simulink model "TBRe19_ECU_1_Brake_Pressure_Conversion"  (R2017b)
settings: Solver=FixedStepDiscrete  StartTime=0.0  StopTime=inf  FixedStep=0.0001  RelTol=1e-3
PostLoadFcn:
  | model_init();
libraries: simulink x17
(part 7 of 7)

== system TBRe19_ECU_1_Brake_Pressure_Conversion/MainTask/Vehicle_Functionality_Layer/Drive_Function/Throttle_withBoost ==
  note: Throttle to torque map -
      | - What percentage of max torque to request based on throttle
      | - Needs adjusting (possibly)
  note: Max torque request to motor (at 100% throttle) under normal operation
  note: Max torque request to motor (at 100% throttle) in boost mode
  note: only acts on down press
  Throttle : Inport
  Button : Inport  Port=2
  BoostActive : Switch  Criteria=u2 ~= 0  OutDataTypeStr=int16
  Delay : Delay  DelayLength=1  InitialCondition=0
  Divide1 : Product  Inputs=**
  Divide3 : Product  Inputs=**
  ModeChange : Logic  Operator=XOR  AllPortsSameDT=off  OutDataTypeStr=boolean
  NOT : Logic  Operator=NOT  AllPortsSameDT=off  OutDataTypeStr=boolean
  RisingEdgeDet : Logic  AllPortsSameDT=off  OutDataTypeStr=boolean
  Throttle_Torque_Map_% : Lookup_n-D  NumberOfTableDimensions=1  BreakpointsForDimension1=[0,30,75,100]  Table=[0,5,50,100]  ExtrapMethod=Clip  UseLastTableValue=on  InternalRulePriority=Speed  OutDataTypeStr=int16  RndMeth=Simplest  InputSameDT=on
  UsbRx : S-Function  FunctionName=NsiUsb_Rx  Parameters=signame,sigtype,resolution,offset,unite,value,is_trigger  SFunctionDeploymentMode=off  EnableBusSupport=off  mask(MUXlink Usb Rx){signame=Max_Torque_Std, sigtype=Unsigned Byte, resolution=1, offset=0.01, unite=Nm, value=120, is_trigger=off}
      mask prompts: signame "Signal name :"; sigtype "Signal type :"; resolution "Resolution :"; offset "Offset :"; unite "Unit :"; value "Default value :"; is_trigger "Is trigger ?"
      mask help: Receive a frame on the USB Channel.
      mask init:
      | NsiUsb_Rx_InitializationFcn();
      settings: OpenFcn=NsiUsb_Rx_OpenFcn();
      mask Help:
      | eval('block=get_param(gcb, ''RTWdata'');')
      | web([docroot '\toolbox\MUXlink\html\blocks/' block.MUXlink_BlockType '.html'])
      mask Callback signame: NsiUsb_Rx_ApplyFcn(1);
      mask TypeOptions sigtype: Boolean | Signed Byte | Unsigned Byte | Signed Word | Unsigned Word | Signed Double Word | Unsigned Double Word | Single Float | Double Float
      mask Callback sigtype: NsiUsb_Rx_ApplyFcn(2);
      mask Callback resolution: NsiUsb_Rx_ApplyFcn(3);
      mask Callback offset: NsiUsb_Rx_ApplyFcn(4);
      mask Callback unite: NsiUsb_Rx_ApplyFcn(5);
      mask Callback value: NsiUsb_Rx_ApplyFcn(6);
      mask Callback is_trigger: NsiUsb_Rx_ApplyFcn(7);
      mask Display: image(imread('nsi.bmp'));text(0.5, 0.2, 'USB Rx', 'horizontalAlignment', 'center', 'verticalAlignment', 'base');plot([0.05 0.05 0.05 0.05 0.05 0.05 0.05 0.05 0.05 0.05]);port_label('output',1, 'Max_Torque_Std');
  UsbRx1 : S-Function  FunctionName=NsiUsb_Rx  Parameters=signame,sigtype,resolution,offset,unite,value,is_trigger  SFunctionDeploymentMode=off  EnableBusSupport=off  mask(MUXlink Usb Rx){signame=Max_Torque_Boost, sigtype=Unsigned Byte, resolution=1, offset=0.01, unite=Nm, value=240, is_trigger=off}
      mask prompts: signame "Signal name :"; sigtype "Signal type :"; resolution "Resolution :"; offset "Offset :"; unite "Unit :"; value "Default value :"; is_trigger "Is trigger ?"
      mask help: Receive a frame on the USB Channel.
      mask init:
      | NsiUsb_Rx_InitializationFcn();
      settings: OpenFcn=NsiUsb_Rx_OpenFcn();
      mask Help:
      | eval('block=get_param(gcb, ''RTWdata'');')
      | web([docroot '\toolbox\MUXlink\html\blocks/' block.MUXlink_BlockType '.html'])
      mask Callback signame: NsiUsb_Rx_ApplyFcn(1);
      mask TypeOptions sigtype: Boolean | Signed Byte | Unsigned Byte | Signed Word | Unsigned Word | Signed Double Word | Unsigned Double Word | Single Float | Double Float
      mask Callback sigtype: NsiUsb_Rx_ApplyFcn(2);
      mask Callback resolution: NsiUsb_Rx_ApplyFcn(3);
      mask Callback offset: NsiUsb_Rx_ApplyFcn(4);
      mask Callback unite: NsiUsb_Rx_ApplyFcn(5);
      mask Callback value: NsiUsb_Rx_ApplyFcn(6);
      mask Callback is_trigger: NsiUsb_Rx_ApplyFcn(7);
      mask Display: image(imread('nsi.bmp'));text(0.5, 0.2, 'USB Rx', 'horizontalAlignment', 'center', 'verticalAlignment', 'base');plot([0.05 0.05 0.05 0.05 0.05 0.05 0.05 0.05 0.05 0.05]);port_label('output',1, 'Max_Torque_Boost');
  prvCheck : Delay  DelayLength=1  InitialCondition=0
  Throttle_Request : Outport
  Boost_On : Outport  Port=2
  wires:
  ModeChange/1 -> Boost_On/1, BoostActive/2, Delay/1
  Throttle/1 -> Throttle_Torque_Map_%/1
  Throttle_Torque_Map_%/1 -> Divide3/1, Divide1/2  "Throttle_Request"
  Divide3/1 -> BoostActive/3
  BoostActive/1 -> Throttle_Request/1
  UsbRx1/1 -> Divide1/1
  Divide1/1 -> BoostActive/1
  UsbRx/1 -> Divide3/2
  RisingEdgeDet/1 -> ModeChange/1
  NOT/1 -> RisingEdgeDet/2
  prvCheck/1 -> NOT/1
  Delay/1 -> ModeChange/2
  Button/1 -> RisingEdgeDet/1, prvCheck/1

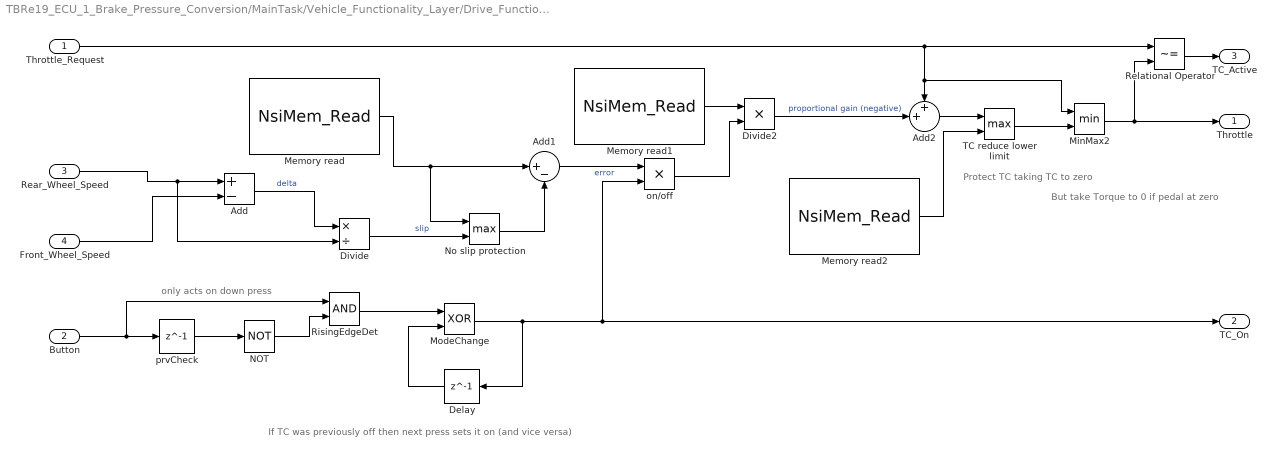
== system TBRe19_ECU_1_Brake_Pressure_Conversion/MainTask/Vehicle_Functionality_Layer/Drive_Function/Traction Control ==
  note: But take Torque to 0 if pedal at zero
  note: Protect TC taking TC to zero
  note: If TC was previously off then next press sets it on (and vice versa)
  note: only acts on down press
  Throttle_Request : Inport
  "Button " : Inport  Port=2
  Rear_Wheel_Speed : Inport  Port=3
  Front_Wheel_Speed : Inport  Port=4
  Add : Sum  Inputs=+-
  Add1 : Sum  Inputs=|+-
  Add2 : Sum  Inputs=++|
  Delay : Delay  DelayLength=1  InitialCondition=0
  Divide : Product  Inputs=*/
  Divide2 : Product  Inputs=**
  Memory read : S-Function  FunctionName=NsiMem_Read  Parameters=name_var,type_var,size_var,tunable_var  SFunctionDeploymentMode=off  EnableBusSupport=off  mask(Memory read){name_var=Target_Slip_Ratio, type_var=Single Float, size_var=1, tunable_var=on}
      mask prompts: name_var "Variable name :"; type_var "Type :"; size_var "Dim of table :"; tunable_var "Is Tunable By USB?"
      mask help: Reads current value of variable memory declared in the configurator block in calibration page.
      mask init:
      | NsiMem_Read_InitializationFcn();
      settings: OpenFcn=NsiMem_Read_OpenFcn();
      mask Help:
      | eval('block=get_param(gcb, ''RTWdata'');')
      | web([docroot '\toolbox\MUXlink\html\blocks/' block.MUXlink_BlockType '.html'])
      mask TypeOptions name_var: Gearing_Ratio | Wheel_Size | Brake1_High | Brake2_High | Accel1_High | Accel2_High | Brake1_Low | Brake2_Low | Accel1_Low | Accel2_Low | Max_Torque_Std | Max_Torque_Boost | MCU_Ignition | LV_Low_Voltage_Warning | MCUMotor_Temp_Warning | Target_Slip_Ratio | TC_P_Gain | MinTC_Torque | Max_Regen
      mask Callback name_var: NsiMem_Read_ApplyFcn(1);
      mask TypeOptions type_var: Boolean | Signed Byte | Unsigned Byte | Signed Word | Unsigned Word | Signed Double Word | Unsigned Double Word | Single Float | Double Float
      mask Callback type_var: NsiMem_Read_ApplyFcn(2);
      mask Callback size_var: NsiMem_Read_ApplyFcn(3);
      mask Callback tunable_var: NsiMem_Read_ApplyFcn(4);
      mask Display: image(imread('nsi.bmp'));text(0.5, 0.35, 'Target_Slip_Ratio', 'horizontalAlignment', 'center', 'verticalAlignment', 'base');plot([0.05 0.05 0.05 0.05 0.05 0.05 0.05 0.05 0.05 0.05]);port_label('output', 1, 'Read');
  Memory read1 : S-Function  FunctionName=NsiMem_Read  Parameters=name_var,type_var,size_var,tunable_var  SFunctionDeploymentMode=off  EnableBusSupport=off  mask(Memory read){name_var=TC_P_Gain, type_var=Unsigned Byte, size_var=1, tunable_var=on}
      mask prompts: name_var "Variable name :"; type_var "Type :"; size_var "Dim of table :"; tunable_var "Is Tunable By USB?"
      mask help: Reads current value of variable memory declared in the configurator block in calibration page.
      mask init:
      | NsiMem_Read_InitializationFcn();
      settings: OpenFcn=NsiMem_Read_OpenFcn();
      mask Help:
      | eval('block=get_param(gcb, ''RTWdata'');')
      | web([docroot '\toolbox\MUXlink\html\blocks/' block.MUXlink_BlockType '.html'])
      mask TypeOptions name_var: Gearing_Ratio | Wheel_Size | Brake1_High | Brake2_High | Accel1_High | Accel2_High | Brake1_Low | Brake2_Low | Accel1_Low | Accel2_Low | Max_Torque_Std | Max_Torque_Boost | MCU_Ignition | LV_Low_Voltage_Warning | MCUMotor_Temp_Warning | Target_Slip_Ratio | TC_P_Gain | MinTC_Torque | Max_Regen
      mask Callback name_var: NsiMem_Read_ApplyFcn(1);
      mask TypeOptions type_var: Boolean | Signed Byte | Unsigned Byte | Signed Word | Unsigned Word | Signed Double Word | Unsigned Double Word | Single Float | Double Float
      mask Callback type_var: NsiMem_Read_ApplyFcn(2);
      mask Callback size_var: NsiMem_Read_ApplyFcn(3);
      mask Callback tunable_var: NsiMem_Read_ApplyFcn(4);
      mask Display: image(imread('nsi.bmp'));text(0.5, 0.35, 'TC_P_Gain', 'horizontalAlignment', 'center', 'verticalAlignment', 'base');plot([0.05 0.05 0.05 0.05 0.05 0.05 0.05 0.05 0.05 0.05]);port_label('output', 1, 'Read');
  Memory read2 : S-Function  FunctionName=NsiMem_Read  Parameters=name_var,type_var,size_var,tunable_var  SFunctionDeploymentMode=off  EnableBusSupport=off  mask(Memory read){name_var=MinTC_Torque, type_var=Unsigned Byte, size_var=1, tunable_var=on}
      mask prompts: name_var "Variable name :"; type_var "Type :"; size_var "Dim of table :"; tunable_var "Is Tunable By USB?"
      mask help: Reads current value of variable memory declared in the configurator block in calibration page.
      mask init:
      | NsiMem_Read_InitializationFcn();
      settings: OpenFcn=NsiMem_Read_OpenFcn();
      mask Help:
      | eval('block=get_param(gcb, ''RTWdata'');')
      | web([docroot '\toolbox\MUXlink\html\blocks/' block.MUXlink_BlockType '.html'])
      mask TypeOptions name_var: Gearing_Ratio | Wheel_Size | Brake1_High | Brake2_High | Accel1_High | Accel2_High | Brake1_Low | Brake2_Low | Accel1_Low | Accel2_Low | Max_Torque_Std | Max_Torque_Boost | MCU_Ignition | LV_Low_Voltage_Warning | MCUMotor_Temp_Warning | Target_Slip_Ratio | TC_P_Gain | MinTC_Torque | Max_Regen
      mask Callback name_var: NsiMem_Read_ApplyFcn(1);
      mask TypeOptions type_var: Boolean | Signed Byte | Unsigned Byte | Signed Word | Unsigned Word | Signed Double Word | Unsigned Double Word | Single Float | Double Float
      mask Callback type_var: NsiMem_Read_ApplyFcn(2);
      mask Callback size_var: NsiMem_Read_ApplyFcn(3);
      mask Callback tunable_var: NsiMem_Read_ApplyFcn(4);
      mask Display: image(imread('nsi.bmp'));text(0.5, 0.35, 'MinTC_Torque', 'horizontalAlignment', 'center', 'verticalAlignment', 'base');plot([0.05 0.05 0.05 0.05 0.05 0.05 0.05 0.05 0.05 0.05]);port_label('output', 1, 'Read');
  MinMax2 : MinMax  Inputs=2
  ModeChange : Logic  Operator=XOR  AllPortsSameDT=off  OutDataTypeStr=boolean
  NOT : Logic  Operator=NOT  AllPortsSameDT=off  OutDataTypeStr=boolean
  No slip protection : MinMax  Function=max  Inputs=2
  Relational Operator : RelationalOperator  Operator=~=  OutDataTypeStr=boolean  RndMeth=Simplest
  RisingEdgeDet : Logic  AllPortsSameDT=off  OutDataTypeStr=boolean
  TC reduce lower limit : MinMax  Function=max  Inputs=2
  on/off : Product  Inputs=**
  prvCheck : Delay  DelayLength=1  InitialCondition=0
  Throttle : Outport
  TC_On : Outport  Port=2
  TC_Active : Outport  Port=3
  wires:
  Rear_Wheel_Speed/1 -> Divide/2, Add/1
  Front_Wheel_Speed/1 -> Add/2
  Add/1 -> Divide/1  "delta"
  Divide/1 -> No slip protection/2  "slip"
  No slip protection/1 -> Add1/2
  Memory read/1 -> No slip protection/1, Add1/1
  Add1/1 -> on/off/1  "error"
  on/off/1 -> Divide2/2
  Memory read1/1 -> Divide2/1
  Divide2/1 -> Add2/2  "proportional gain (negative)"
  Throttle_Request/1 -> Relational Operator/1, MinMax2/1, Add2/1
  Add2/1 -> TC reduce lower limit/1
  NOT/1 -> RisingEdgeDet/2
  Delay/1 -> ModeChange/2
  ModeChange/1 -> on/off/2, TC_On/1, Delay/1
  prvCheck/1 -> NOT/1
  "Button "/1 -> RisingEdgeDet/1, prvCheck/1
  RisingEdgeDet/1 -> ModeChange/1
  TC reduce lower limit/1 -> MinMax2/2
  Memory read2/1 -> TC reduce lower limit/2
  MinMax2/1 -> Relational Operator/2, Throttle/1
  Relational Operator/1 -> TC_Active/1

== system TBRe19_ECU_1_Brake_Pressure_Conversion/MainTask/Vehicle_Functionality_Layer/Vehicle_Operation_Mode/TSS ==
  note: This was the old code
  note: This is checking that AIRLow has closed before being allowed to go RTD
  note: This block gets instant pack voltage from BMS, MCU voltage from MCU
      |
      | If MCU is within 90% of Accy voltage then TSS is true
      |
      | Also needs Accy and MCU to be higher than 200
  note: MCU_Link_Voltage = double(MCU_Link_Voltage);
      |
      | Threshold = 0.90*Pack_Voltage;
      | %Added Check for voltage above 60V so precharge is not open when car turns
      | %on or no accumilator in car
      |
      | if(((MCU_Link_Voltage/10) >= Threshold) && (MCU_Link_Voltage >= 60))
      |     Pre_Charge_Hold = true;
      | else
      |     Pre_Charge_Hold = false;
      | end
  PrePL_Data : Inport
  Accy_Has_Voltage : simulink/Logic and Bit Operations/Compare To Constant  relop=>=  const=150  OutDataTypeStr=boolean
  Add : Sum  Inputs=-+  OutDataTypeStr=int16
  Bus Selector : BusSelector  OutputSignals=DAL_Data.DAL_CAN.DAL_BMSCAN.Instant_Pack_Voltage,DAL_Data.DAL_CAN.DAL_MCUCAN.MCU_Voltage,DAL_Data.DAL_Hardwired.AIRLow
  In_threshold : simulink/Logic and Bit Operations/Compare To Zero  relop=>  OutDataTypeStr=boolean
  MCU_Has_Voltage : simulink/Logic and Bit Operations/Compare To Constant  relop=>=  const=150  OutDataTypeStr=boolean
  Product : Product  Inputs=**  OutDataTypeStr=uint16
  StartUp : Logic  Inputs=3  AllPortsSameDT=off  OutDataTypeStr=boolean
  Threshold_Level : Constant  Value=0.9
  TS_StartUp : Outport
  wires:
  PrePL_Data/1 -> Bus Selector/1
  Bus Selector/1 -> Product/1, Accy_Has_Voltage/1  "<Instant_Pack_Voltage>"
  Threshold_Level/1 -> Product/2
  Product/1 -> Add/1
  Add/1 -> In_threshold/1  "Vdiff"
  In_threshold/1 -> StartUp/2
  MCU_Has_Voltage/1 -> StartUp/3
  StartUp/1 -> TS_StartUp/1  "TSS"
  Bus Selector/2 -> MCU_Has_Voltage/1, Add/2  "<MCU_Voltage>"
  Accy_Has_Voltage/1 -> StartUp/1
  Bus Selector/3 -> ?  "<AIRLow>"

== system TBRe19_ECU_1_Brake_Pressure_Conversion/MainTask/Pre_Processing_Layer/Pedal_Box/Voltage_to_% Conversion/Calibrate ==
  PedalMax : Inport
  PedalMin : Inport  Port=2
  Voltage : Inport  Port=3
  Add : Sum  Inputs=+-
  Add1 : Sum  Inputs=-+
  Constant : Constant  Value=100  OutDataTypeStr=double
  Data Type Conversion3 : DataTypeConversion  OutDataTypeStr=double
  Data Type Conversion4 : DataTypeConversion  OutDataTypeStr=double
  Divide : Product  Inputs=*/*  OutDataTypeStr=double
  MinMax : MinMax  Inputs=2  OutDataTypeStr=uint16
  MinMax5 : MinMax  Function=max  Inputs=2  OutDataTypeStr=uint16
  Percentage : Outport
  wires:
  PedalMin/1 -> Add/2, Add1/1, MinMax5/1
  PedalMax/1 -> Add/1
  Add1/1 -> Data Type Conversion4/1
  Voltage/1 -> MinMax5/2
  Constant/1 -> Divide/1, MinMax/1
  Data Type Conversion3/1 -> Divide/2
  Add/1 -> Data Type Conversion3/1
  Data Type Conversion4/1 -> Divide/3
  Divide/1 -> MinMax/2
  MinMax/1 -> Percentage/1
  MinMax5/1 -> Add1/2

== system TBRe19_ECU_1_Brake_Pressure_Conversion/MainTask/Pre_Processing_Layer/Pedal_Box/Voltage_to_% Conversion/Calibrate1 ==
  PedalMax : Inport
  PedalMin : Inport  Port=2
  Voltage : Inport  Port=3
  Add : Sum  Inputs=+-
  Add1 : Sum  Inputs=-+
  Constant : Constant  Value=100  OutDataTypeStr=double
  Data Type Conversion3 : DataTypeConversion  OutDataTypeStr=double
  Data Type Conversion4 : DataTypeConversion  OutDataTypeStr=double
  Divide : Product  Inputs=*/*  OutDataTypeStr=double
  MinMax : MinMax  Inputs=2  OutDataTypeStr=uint16
  MinMax5 : MinMax  Function=max  Inputs=2  OutDataTypeStr=uint16
  Percentage : Outport
  wires:
  PedalMin/1 -> Add/2, Add1/1, MinMax5/1
  PedalMax/1 -> Add/1
  Add1/1 -> Data Type Conversion4/1
  Voltage/1 -> MinMax5/2
  Constant/1 -> Divide/1, MinMax/1
  Data Type Conversion3/1 -> Divide/2
  Add/1 -> Data Type Conversion3/1
  Data Type Conversion4/1 -> Divide/3
  Divide/1 -> MinMax/2
  MinMax/1 -> Percentage/1
  MinMax5/1 -> Add1/2

== system TBRe19_ECU_1_Brake_Pressure_Conversion/MainTask/Pre_Processing_Layer/Pedal_Box/Voltage_to_% Conversion/Calibrate2 ==
  PedalMax : Inport
  PedalMin : Inport  Port=2
  Voltage : Inport  Port=3
  Add : Sum  Inputs=+-
  Add1 : Sum  Inputs=-+
  Add2 : Sum  Inputs=-+
  Constant : Constant  Value=100  OutDataTypeStr=double
  Data Type Conversion3 : DataTypeConversion  OutDataTypeStr=double
  Data Type Conversion4 : DataTypeConversion  OutDataTypeStr=double
  Divide : Product  Inputs=*/*  OutDataTypeStr=double
  Divide1 : Product  Inputs=**  OutDataTypeStr=double
  Gain : Gain  Gain=0.0145038
  Memory read9 : S-Function  FunctionName=NsiMem_Read  Parameters=name_var,type_var,size_var,tunable_var  SFunctionDeploymentMode=off  EnableBusSupport=off  mask(Memory read){name_var=Brake1_Pressure_Scaling, type_var=Signed Byte, size_var=1, tunable_var=on}
      mask prompts: name_var "Variable name :"; type_var "Type :"; size_var "Dim of table :"; tunable_var "Is Tunable By USB?"
      mask help: Reads current value of variable memory declared in the configurator block in calibration page.
      mask init:
      | NsiMem_Read_InitializationFcn();
      settings: OpenFcn=NsiMem_Read_OpenFcn();
      mask Help:
      | eval('block=get_param(gcb, ''RTWdata'');')
      | web([docroot '\toolbox\MUXlink\html\blocks/' block.MUXlink_BlockType '.html'])
      mask TypeOptions name_var: Gearing_Ratio | Wheel_Size | Brake1_High | Brake2_High | Throttle1_High | Throttle2_High | Brake1_Low | Brake2_Low | Throttle1_Low | Throttle2_Low | Max_Torque_Std | Max_Torque_Boost | MCU_Ignition | LV_Low_Voltage_Warning | MCUMotor_Temp_Warning | Target_Slip_Ratio | TC_P_Gain | MinTC_Torque | Max_Regen | Throttle_Active_Threshold | Brake_Active_Threshold | INV_Torque_limit | INV_Speed_Limit_Fwd | INV_Speed_limit_Rev | INV_DC_Link_Target | INV_DC_Link_Regen_Imax | INV_DC_Link_Discharge_Imax | INV_Regen_Torque_Limit | INV_Id_Debug | INV_Iq_debug | Init_System_Start | Init_System_end | Brake1_Pressure_Scaling | Brake2_Pressure_Scaling
      mask Callback name_var: NsiMem_Read_ApplyFcn(1);
      mask TypeOptions type_var: Boolean | Signed Byte | Unsigned Byte | Signed Word | Unsigned Word | Signed Double Word | Unsigned Double Word | Single Float | Double Float
      mask Callback type_var: NsiMem_Read_ApplyFcn(2);
      mask Callback size_var: NsiMem_Read_ApplyFcn(3);
      mask Callback tunable_var: NsiMem_Read_ApplyFcn(4);
      mask Display: image(imread('nsi.bmp'));text(0.5, 0.35, 'Brake1_Pressure_Scaling', 'horizontalAlignment', 'center', 'verticalAlignment', 'base');plot([0.05 0.05 0.05 0.05 0.05 0.05 0.05 0.05 0.05 0.05]);port_label('output', 1, 'Read');
  MinMax : MinMax  Inputs=2  OutDataTypeStr=uint16
  MinMax5 : MinMax  Function=max  Inputs=2  OutDataTypeStr=uint16
  UsbTx1 : S-Function  FunctionName=NsiUsb_Tx  Parameters=signame,resolution,offset,unite  SFunctionDeploymentMode=off  EnableBusSupport=off  mask(MUXlink Usb Tx){signame=Brake1PSI, resolution=1, offset=0, unite=PSI}
      mask prompts: signame "Signal name ?"; resolution "Resolution ?"; offset "Offset ?"; unite "Unit ?"
      mask help: Transmit a frame on the USB Channel.
      mask init:
      | NsiUsb_Tx_InitializationFcn();
      settings: OpenFcn=NsiUsb_Tx_OpenFcn();
      mask Help:
      | eval('block=get_param(gcb, ''RTWdata'');')
      | web([docroot '\toolbox\MUXlink\html\blocks/' block.MUXlink_BlockType '.html'])
      mask Callback signame: NsiUsb_Tx_ApplyFcn(1);
      mask Callback resolution: NsiUsb_Tx_ApplyFcn(2);
      mask Callback offset: NsiUsb_Tx_ApplyFcn(3);
      mask Callback unite: NsiUsb_Tx_ApplyFcn(4);
      mask Display: image(imread('nsi.bmp'));text(0.5, 0.2, 'USB Tx', 'horizontalAlignment', 'center', 'verticalAlignment', 'base');plot([0.05 0.05 0.05 0.05 0.05 0.05 0.05 0.05 0.05 0.05]);port_label('input',1, 'Brake1PSI');
  UsbTx5 : S-Function  FunctionName=NsiUsb_Tx  Parameters=signame,resolution,offset,unite  SFunctionDeploymentMode=off  EnableBusSupport=off  mask(MUXlink Usb Tx){signame=Brake1mBar, resolution=1, offset=0, unite=mBar}
      mask prompts: signame "Signal name ?"; resolution "Resolution ?"; offset "Offset ?"; unite "Unit ?"
      mask help: Transmit a frame on the USB Channel.
      mask init:
      | NsiUsb_Tx_InitializationFcn();
      settings: OpenFcn=NsiUsb_Tx_OpenFcn();
      mask Help:
      | eval('block=get_param(gcb, ''RTWdata'');')
      | web([docroot '\toolbox\MUXlink\html\blocks/' block.MUXlink_BlockType '.html'])
      mask Callback signame: NsiUsb_Tx_ApplyFcn(1);
      mask Callback resolution: NsiUsb_Tx_ApplyFcn(2);
      mask Callback offset: NsiUsb_Tx_ApplyFcn(3);
      mask Callback unite: NsiUsb_Tx_ApplyFcn(4);
      mask Display: image(imread('nsi.bmp'));text(0.5, 0.2, 'USB Tx', 'horizontalAlignment', 'center', 'verticalAlignment', 'base');plot([0.05 0.05 0.05 0.05 0.05 0.05 0.05 0.05 0.05 0.05]);port_label('input',1, 'Brake1mBar');
  Percentage : Outport
  wires:
  PedalMin/1 -> Add2/1, MinMax5/1, Add1/1, Add/2
  PedalMax/1 -> Add/1
  Add1/1 -> Data Type Conversion4/1
  Voltage/1 -> Add2/2, MinMax5/2
  Constant/1 -> Divide/1, MinMax/1
  Data Type Conversion3/1 -> Divide/2
  Add/1 -> Data Type Conversion3/1
  Data Type Conversion4/1 -> Divide/3
  Divide/1 -> MinMax/2
  MinMax/1 -> Percentage/1
  MinMax5/1 -> Add1/2
  Add2/1 -> Divide1/1
  Memory read9/1 -> Divide1/2
  Gain/1 -> UsbTx1/1
  Divide1/1 -> Gain/1, UsbTx5/1

== system TBRe19_ECU_1_Brake_Pressure_Conversion/MainTask/Pre_Processing_Layer/Pedal_Box/Voltage_to_% Conversion/Calibrate3 ==
  PedalMax : Inport
  PedalMin : Inport  Port=2
  Voltage : Inport  Port=3
  Add : Sum  Inputs=+-
  Add1 : Sum  Inputs=-+
  Add2 : Sum  Inputs=-+
  Constant : Constant  Value=100  OutDataTypeStr=double
  Data Type Conversion3 : DataTypeConversion  OutDataTypeStr=double
  Data Type Conversion4 : DataTypeConversion  OutDataTypeStr=double
  Divide : Product  Inputs=*/*  OutDataTypeStr=double
  Divide1 : Product  Inputs=**  OutDataTypeStr=double
  Gain : Gain  Gain=0.0145038
  Memory read8 : S-Function  FunctionName=NsiMem_Read  Parameters=name_var,type_var,size_var,tunable_var  SFunctionDeploymentMode=off  EnableBusSupport=off  mask(Memory read){name_var=Brake2_Pressure_Scaling, type_var=Signed Byte, size_var=1, tunable_var=on}
      mask prompts: name_var "Variable name :"; type_var "Type :"; size_var "Dim of table :"; tunable_var "Is Tunable By USB?"
      mask help: Reads current value of variable memory declared in the configurator block in calibration page.
      mask init:
      | NsiMem_Read_InitializationFcn();
      settings: OpenFcn=NsiMem_Read_OpenFcn();
      mask Help:
      | eval('block=get_param(gcb, ''RTWdata'');')
      | web([docroot '\toolbox\MUXlink\html\blocks/' block.MUXlink_BlockType '.html'])
      mask TypeOptions name_var: Gearing_Ratio | Wheel_Size | Brake1_High | Brake2_High | Throttle1_High | Throttle2_High | Brake1_Low | Brake2_Low | Throttle1_Low | Throttle2_Low | Max_Torque_Std | Max_Torque_Boost | MCU_Ignition | LV_Low_Voltage_Warning | MCUMotor_Temp_Warning | Target_Slip_Ratio | TC_P_Gain | MinTC_Torque | Max_Regen | Throttle_Active_Threshold | Brake_Active_Threshold | INV_Torque_limit | INV_Speed_Limit_Fwd | INV_Speed_limit_Rev | INV_DC_Link_Target | INV_DC_Link_Regen_Imax | INV_DC_Link_Discharge_Imax | INV_Regen_Torque_Limit | INV_Id_Debug | INV_Iq_debug | Init_System_Start | Init_System_end | Brake1_Pressure_Scaling | Brake2_Pressure_Scaling
      mask Callback name_var: NsiMem_Read_ApplyFcn(1);
      mask TypeOptions type_var: Boolean | Signed Byte | Unsigned Byte | Signed Word | Unsigned Word | Signed Double Word | Unsigned Double Word | Single Float | Double Float
      mask Callback type_var: NsiMem_Read_ApplyFcn(2);
      mask Callback size_var: NsiMem_Read_ApplyFcn(3);
      mask Callback tunable_var: NsiMem_Read_ApplyFcn(4);
      mask Display: image(imread('nsi.bmp'));text(0.5, 0.35, 'Brake2_Pressure_Scaling', 'horizontalAlignment', 'center', 'verticalAlignment', 'base');plot([0.05 0.05 0.05 0.05 0.05 0.05 0.05 0.05 0.05 0.05]);port_label('output', 1, 'Read');
  MinMax : MinMax  Inputs=2  OutDataTypeStr=uint16
  MinMax5 : MinMax  Function=max  Inputs=2  OutDataTypeStr=uint16
  UsbTx1 : S-Function  FunctionName=NsiUsb_Tx  Parameters=signame,resolution,offset,unite  SFunctionDeploymentMode=off  EnableBusSupport=off  mask(MUXlink Usb Tx){signame=Brake2PSI, resolution=1, offset=0, unite=PSI}
      mask prompts: signame "Signal name ?"; resolution "Resolution ?"; offset "Offset ?"; unite "Unit ?"
      mask help: Transmit a frame on the USB Channel.
      mask init:
      | NsiUsb_Tx_InitializationFcn();
      settings: OpenFcn=NsiUsb_Tx_OpenFcn();
      mask Help:
      | eval('block=get_param(gcb, ''RTWdata'');')
      | web([docroot '\toolbox\MUXlink\html\blocks/' block.MUXlink_BlockType '.html'])
      mask Callback signame: NsiUsb_Tx_ApplyFcn(1);
      mask Callback resolution: NsiUsb_Tx_ApplyFcn(2);
      mask Callback offset: NsiUsb_Tx_ApplyFcn(3);
      mask Callback unite: NsiUsb_Tx_ApplyFcn(4);
      mask Display: image(imread('nsi.bmp'));text(0.5, 0.2, 'USB Tx', 'horizontalAlignment', 'center', 'verticalAlignment', 'base');plot([0.05 0.05 0.05 0.05 0.05 0.05 0.05 0.05 0.05 0.05]);port_label('input',1, 'Brake2PSI');
  UsbTx6 : S-Function  FunctionName=NsiUsb_Tx  Parameters=signame,resolution,offset,unite  SFunctionDeploymentMode=off  EnableBusSupport=off  mask(MUXlink Usb Tx){signame=Brake2mBar, resolution=1, offset=0, unite=mBar}
      mask prompts: signame "Signal name ?"; resolution "Resolution ?"; offset "Offset ?"; unite "Unit ?"
      mask help: Transmit a frame on the USB Channel.
      mask init:
      | NsiUsb_Tx_InitializationFcn();
      settings: OpenFcn=NsiUsb_Tx_OpenFcn();
      mask Help:
      | eval('block=get_param(gcb, ''RTWdata'');')
      | web([docroot '\toolbox\MUXlink\html\blocks/' block.MUXlink_BlockType '.html'])
      mask Callback signame: NsiUsb_Tx_ApplyFcn(1);
      mask Callback resolution: NsiUsb_Tx_ApplyFcn(2);
      mask Callback offset: NsiUsb_Tx_ApplyFcn(3);
      mask Callback unite: NsiUsb_Tx_ApplyFcn(4);
      mask Display: image(imread('nsi.bmp'));text(0.5, 0.2, 'USB Tx', 'horizontalAlignment', 'center', 'verticalAlignment', 'base');plot([0.05 0.05 0.05 0.05 0.05 0.05 0.05 0.05 0.05 0.05]);port_label('input',1, 'Brake2mBar');
  Percentage : Outport
  wires:
  PedalMin/1 -> Add2/1, MinMax5/1, Add1/1, Add/2
  PedalMax/1 -> Add/1
  Add1/1 -> Data Type Conversion4/1
  Voltage/1 -> MinMax5/2, Add2/2
  Constant/1 -> Divide/1, MinMax/1
  Data Type Conversion3/1 -> Divide/2
  Add/1 -> Data Type Conversion3/1
  Data Type Conversion4/1 -> Divide/3
  Divide/1 -> MinMax/2
  MinMax/1 -> Percentage/1
  MinMax5/1 -> Add1/2
  Divide1/1 -> Gain/1, UsbTx6/1
  Add2/1 -> Divide1/1
  Memory read8/1 -> Divide1/2
  Gain/1 -> UsbTx1/1

== matlab function TBRe19_ECU_1_Brake_Pressure_Conversion/MainTask/Vehicle_Functionality_Layer/Drive_Function/Regen_Braking1/Torque_Mode ==
  data: Throttle input; Brake input; Torque output; Coast input; Speed input; RegenOk input; RegenBool output
function [Torque, RegenBool]= fcn(Throttle, Brake, Coast,Speed,RegenOk )
%Set Torque depending on drive, coas of braking
Coast = int16(Coast);
RegenBool = false;
if(Throttle > 5)
    %Driving Demand
    Torque = int16(Throttle);
elseif(Throttle <= 5 && Brake  <= 80 && Speed > 1.5 && RegenOk == true)
    %Vehicle is coasting
    Torque = int16(Coast);
    RegenBool = true;
else
    %Safety
    Torque = int16(0);
end

== stateflow chart TBRe19_ECU_1_Brake_Pressure_Conversion/MainTask/Vehicle_Functionality_Layer/Vehicle_Operation_Mode/Operaton_Mode ==
  note: Start here
  state Standby_State
    entry:
    Control_Word = uint8(6); %Off
    MCU_NMT_Mode = uint8(2); %Pre-Operational Mode
    State = 1;
  state Error_State
    entry:
    Control_Word = uint8(6); %Error
    MCU_NMT_Mode = uint8(0); %Stopped Mode
    State = 0;
  note: (ECU errors)
  state RTD_Exit_Debounce
    entry:
    Control_Word = uint8(6); %Off
    MCU_NMT_Mode = uint8(2); %Pre-Operational Mode
    State = 1;
  note: btnRTD is for rules
      | TSS is for our safety
  state Buzzer_State
    entry:
    Control_Word = uint8(3); %Energise
    MCU_NMT_Mode = uint8(2); %Pre-Operational Mode
    State = 2;
  state RTD_State
    entry:
    Control_Word = uint8(5); %ReadyToDrive
    MCU_NMT_Mode = uint8(3); %Operational Mode
    State = 3;
  Standby_State -> Error_State [order 1] : [Error]
  (default) -> Error_State
  Error_State -> Standby_State : [~Error]
  RTD_Exit_Debounce -> Standby_State : after(0.5,sec)
  Standby_State -> Buzzer_State [order 2] : [btnRTD && Brake && ~Throttle && TSS]
  RTD_State -> Error_State [order 1] : [Error]
  Buzzer_State -> Error_State [order 1] : [Error]
  RTD_State -> RTD_Exit_Debounce [order 2] : [btnRTD || ~TSS]
  Buzzer_State -> RTD_State [order 2] : after(1.5,sec)
  data: MCU_NMT_Mode output uint8; Control_Word output uint8; State output uint8; Throttle input boolean; Brake input boolean; btnRTD input boolean; btnRTD_Hold input boolean; Error input boolean; TSS input boolean

== stateflow chart TBRe19_ECU_1_Brake_Pressure_Conversion/MainTask/Post_Processing_Layer/Dash_LEDs/InitLight ==
  state Init
    entry:
    Light = true;
  state Normal
    entry:
    Light = false;
  (default) -> Init
  Init -> Normal : after(2.5,sec)
  data: Light output boolean =true

== stateflow chart TBRe19_ECU_1_Brake_Pressure_Conversion/MainTask/Post_Processing_Layer/Dash_LEDs/Wake_Up ==
  state Init
    entry:
    RTD = true;
    X = false;
    Y = false;
    Z = false;
  state One
    entry:
    RTD = false;
    X = true;
    Y = false;
    Z = false;
  state Two
    entry:
    RTD = false;
    X = false;
    Y = true;
    Z = false;
  state Three
    entry:
    RTD = false;
    X = false;
    Y = false;
    Z = true;
  state Normal
    entry:
    RTD = false;
    X = false;
    Y = false;
    Z = false;
  (default) -> Init
  Init -> One : after(0.5,sec)
  One -> Two : after(0.5,sec)
  Two -> Three : after(0.5, sec)
  Three -> Normal : after(0.5, sec)
  data: RTD output boolean =true; X output boolean =true; Y output boolean =true; Z output boolean =true

== stateflow chart TBRe19_ECU_1_Brake_Pressure_Conversion/MainTask/Post_Processing_Layer/Dash_LEDs/Flashy ==
  state Init
    entry:
    Light = true;
  state Normal
    entry:
    Light = false;
  (default) -> Init
  Init -> Normal : after(0.5,sec)
  Normal -> Init : after(0.5,sec)
  data: Light output boolean =true

== stateflow chart TBRe19_ECU_1_Brake_Pressure_Conversion/MainTask/Comms_And_Data_Output_Layer/Hardwired_Ouputs/Operation_Mode ==
  note: Start here
  state Operating_State
    entry:
    Operating_State = 0; %Normal Operation
  state Startup_State
    entry:
    Operating_State = 1; %Reset
  (default) -> Startup_State
  Startup_State -> Operating_State : after(1.5,sec)
  data: Operating_State output boolean

== stateflow chart TBRe19_ECU_1_Brake_Pressure_Conversion/MainTask/Post_Processing_Layer/Dash_LEDs/Flashy1 ==
  state Init
    entry:
    Light = true;
  state Normal
    entry:
    Light = false;
  (default) -> Init
  Init -> Normal : after(0.33,sec)
  Normal -> Init : after(0.33,sec)
  data: Light output boolean =true

== stateflow chart TBRe19_ECU_1_Brake_Pressure_Conversion/MainTask/Post_Processing_Layer/Hardwired_Peripherals/Operation_Mode1 ==
  note: Start here
  state Operating_State
    entry:
    Ignition = 0; %Off
  state Startup_State
    entry:
    Ignition = 1; %Default
  (default) -> Startup_State
  Startup_State -> Operating_State : [Ignition_Switch]
  Operating_State -> Startup_State : after(1.5,sec)
  data: Ignition_Switch input boolean; Ignition output boolean

== matlab function TBRe19_ECU_1_Brake_Pressure_Conversion/MainTask/Vehicle_Functionality_Layer/Drive_Function/Regen_Braking_Old/Torque_Mode ==
  data: Throttle input; Torque output; Brake input; Coast input; Speed input; RegenOk input; RegenBool output
function [Torque, RegenBool]= fcn(Throttle, Brake, Coast,Speed,RegenOk )
%Set Torque depending on drive, coas of braking
Coast = int16(Coast);


if(Throttle > 0)
    %Driving Demand
    Torque = int16(Throttle);
elseif(Throttle == 0 && Brake  == 0)
    %Vehicle is coasting
    Torque = int16(Coast);
elseif(Brake > 0)
    %Vehicle is braking
    Torque = int16(Brake);
else
    %Safety
    Torque = int16(0);
end

if (RegenOk == false && Torque < 0)
    Torque  = int16(0);
elseif (Speed < 1.5 && Torque < 0) %5km/h rule is 1.4 m/s
    Torque  = int16(0);
    %Don't regen when vehicle is stationary 
else
    Torque = int16(Torque);
    %nothing
end


if(Torque < 0)
    RegenBool = true;
else
    RegenBool = false;
end

== matlab function TBRe19_ECU_1_Brake_Pressure_Conversion/MainTask/Pre_Processing_Layer/Pedal_Box/Sensor Plausibility/Sensor_Diag ==
  data: TV_1 input; Pedal_Sensor_Fail output; TV_2 input; BV_POT input; TV1_Out output; TV2_Out output; BV_1 input; BVPot_Out output; BV_2 input; BV1_Out output; BV2_Out output
function [Pedal_Sensor_Fail,TV1_Out,TV2_Out,BVPot_Out, BV1_Out, BV2_Out ] = Sensor_Diagnostics(TV_1,TV_2,BV_POT , BV_1, BV_2)
%Checks whether the throttle sensors are in their calibrated range

%Initialisation of throttle outputs, default low 
TV1_Out=uint16(0);
TV2_Out=uint16(0);
BVPot_Out=uint16(0);
BV1_Out=uint16(0);
BV2_Out=uint16(0);

Pedal_Sensor_Fail = uint8(0);

if (TV_1>5000 || TV_1<000) %if V1 out of normal range
    Pedal_Sensor_Fail = Pedal_Sensor_Fail + uint8(1);
   
end

if (TV_2>5000 || TV_2<0000) %if V2 out of normal range
    Pedal_Sensor_Fail = Pedal_Sensor_Fail + uint8(2);
end   

if (BV_POT>5000 || BV_POT<0) %if brake out of normal range
    Pedal_Sensor_Fail = Pedal_Sensor_Fail + uint8(4);
  
end

if (BV_POT>5000 || BV_POT<0) %if brake out of normal range
    Pedal_Sensor_Fail = Pedal_Sensor_Fail + uint8(8);
  
end

if (BV_POT>5000 || BV_POT<0) %if brake out of normal range
    Pedal_Sensor_Fail = Pedal_Sensor_Fail + uint8(16);
  
end

if(Pedal_Sensor_Fail == 0) %if no error pass voltages to pedal checks
    TV1_Out=uint16(TV_1);
    TV2_Out=uint16(TV_2);
    BVPot_Out=uint16(BV_POT);
    BV1_Out = uint16(BV_1);
    BV2_Out = uint16(BV_2);
end
